simulink model "a1_ex2_sim2"  (R2023a)
settings: Solver=FixedStepAuto  StartTime=0.0  StopTime=30  FixedStep=Ts  RelTol=1e-3
InitFcn:
  | a1_ex2_sim_init
values from neighbouring files (symbols this model uses):
  filter_coeff_bp = firpm(n_bp,fo_bp,ao_bp,w_bp)    [a1_ex2_sim_init.m]
  filter_coeff_lp = firpm(n_lp,fo_lp,ao_lp,w_lp)    [a1_ex2_sim_init.m]
  R = [cos(theta) -sin(theta) 0 ... (first row only)    [a1_ex2_sim_init.m]
  rate_limit_falling = -2    [a1_ex2_sim_init.m]
  rate_limit_rising = 2    [a1_ex2_sim_init.m]
  th1_biceps_left = 0.09    [a1_ex2_sim_init.m]
  th1_biceps_right = 0.09    [a1_ex2_sim_init.m]
  th1_trapezius_left = 0.055    [a1_ex2_sim_init.m]
  th1_trapezius_right = 0.08    [a1_ex2_sim_init.m]
  Ts = 1e-3    (= 0.001)    [a1_ex2_sim_init.m]
libraries: vrlib x1
settings Model: Creator=davide  LastModifiedBy=davide

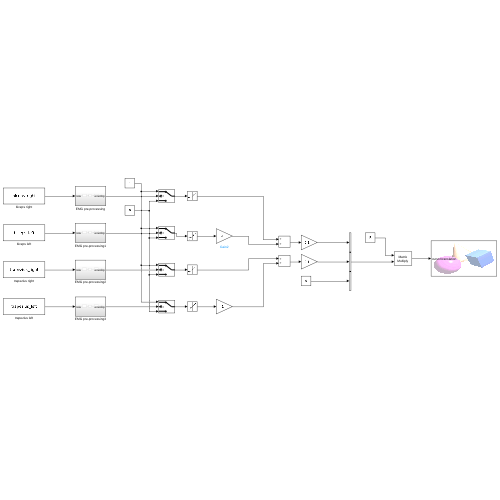
[thumbnail: Simulink's stored preview of the top-level diagram]
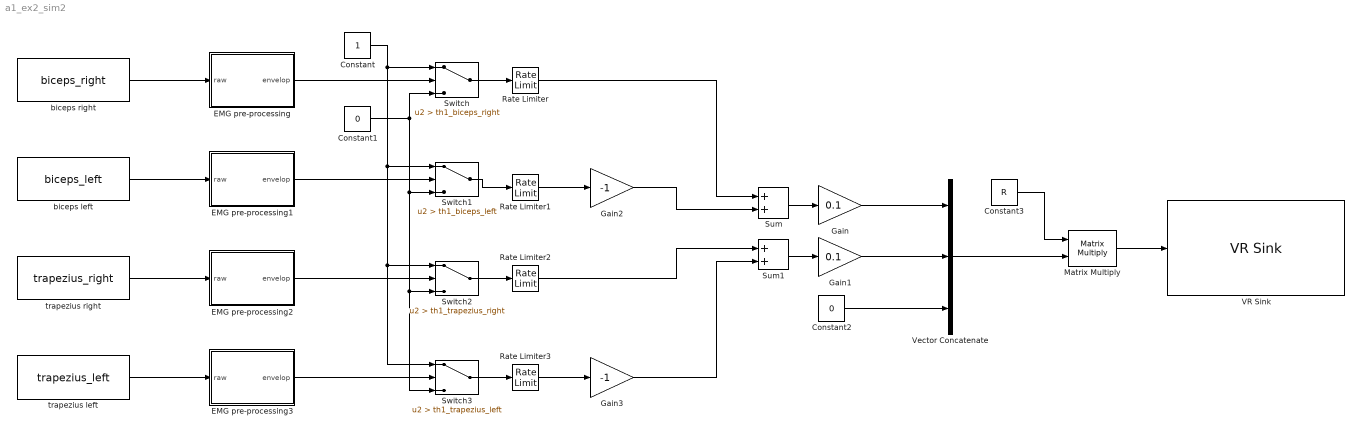
== system a1_ex2_sim2 ==
  Constant : Constant
  Constant1 : Constant  Value=0
  Constant2 : Constant  Value=0
  Constant3 : Constant  Value=R  VectorParams1D=off
  EMG pre-processing : Subsystem
  EMG pre-processing1 : Subsystem
  EMG pre-processing2 : Subsystem
  EMG pre-processing3 : Subsystem
  Gain : Gain  Gain=0.1
  Gain1 : Gain  Gain=0.1
  Gain2 : Gain  Gain=-1
  Gain3 : Gain  Gain=-1
  Matrix Multiply : Product  Multiplication=Matrix(*)
  Rate Limiter{,1..3} (4 alike) : RateLimiter  RisingSlewLimit=rate_limit_rising  FallingSlewLimit=rate_limit_falling  SampleTimeMode=inherited
  Sum : Sum
  Sum1 : Sum
  Switch : Switch  Criteria=u2 > Threshold  Threshold=th1_biceps_right  SaturateOnIntegerOverflow=off  InputSameDT=off
  Switch1 : Switch  Criteria=u2 > Threshold  Threshold=th1_biceps_left  SaturateOnIntegerOverflow=off  InputSameDT=off
  Switch2 : Switch  Criteria=u2 > Threshold  Threshold=th1_trapezius_right  SaturateOnIntegerOverflow=off  InputSameDT=off
  Switch3 : Switch  Criteria=u2 > Threshold  Threshold=th1_trapezius_left  SaturateOnIntegerOverflow=off  InputSameDT=off
  VR Sink : vrlib/VR Sink  InstantiateOnLoad=on  SampleTime=0.1  ViewEnable=on  RemoteChange=off  RemoteView=off  FieldsWritten=cursor.translation.3.1.1.double  WorldFileName=es2_emg/8_palline_color.wrl  AutoView=off  VideoDimensions=[]  AllowVariableSize=off
  Vector Concatenate : Concatenate  NumInputs=3
  biceps left : FromWorkspace  VariableName=biceps_left  OutDataTypeStr=double  SampleTime=Ts
  biceps right : FromWorkspace  VariableName=biceps_right  OutDataTypeStr=double  SampleTime=Ts
  trapezius left : FromWorkspace  VariableName=trapezius_left  OutDataTypeStr=double  SampleTime=Ts
  trapezius right : FromWorkspace  VariableName=trapezius_right  OutDataTypeStr=double  SampleTime=Ts
  wires:
  biceps right/1 -> EMG pre-processing/1(raw)
  biceps left/1 -> EMG pre-processing1/1(raw)
  trapezius right/1 -> EMG pre-processing2/1(raw)
  trapezius left/1 -> EMG pre-processing3/1(raw)
  EMG pre-processing/1(envelop) -> Switch/2
  Constant/1 -> Switch2/1, Switch3/1, Switch1/1, Switch/1
  Constant1/1 -> Switch3/3, Switch2/3, Switch1/3, Switch/3
  Switch/1 -> Rate Limiter/1
  Switch1/1 -> Rate Limiter1/1
  EMG pre-processing1/1(envelop) -> Switch1/2
  EMG pre-processing2/1(envelop) -> Switch2/2
  Switch2/1 -> Rate Limiter2/1
  Switch3/1 -> Rate Limiter3/1
  EMG pre-processing3/1(envelop) -> Switch3/2
  Rate Limiter1/1 -> Gain2/1
  Rate Limiter2/1 -> Sum1/1
  Rate Limiter3/1 -> Gain3/1
  Rate Limiter/1 -> Sum/1
  Gain2/1 -> Sum/2
  Sum/1 -> Gain/1
  Sum1/1 -> Gain1/1
  Gain3/1 -> Sum1/2
  Gain/1 -> Vector Concatenate/1
  Gain1/1 -> Vector Concatenate/2
  Constant3/1 -> Matrix Multiply/1
  Constant2/1 -> Vector Concatenate/3
  Vector Concatenate/1 -> Matrix Multiply/2
  Matrix Multiply/1 -> VR Sink/1

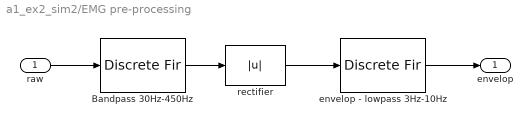
== system a1_ex2_sim2/EMG pre-processing ==
  raw : Inport
  Bandpass 30Hz-450Hz : DiscreteFir  Coefficients=filter_coeff_bp  InputProcessing=Columns as channels (frame based)  SampleTime=Ts
  envelop - lowpass 3Hz-10Hz : DiscreteFir  Coefficients=filter_coeff_lp  InputProcessing=Columns as channels (frame based)  SampleTime=Ts
  rectifier : Abs  SaturateOnIntegerOverflow=off
  envelop : Outport
  wires:
  Bandpass 30Hz-450Hz/1 -> rectifier/1
  rectifier/1 -> envelop - lowpass 3Hz-10Hz/1
  envelop - lowpass 3Hz-10Hz/1 -> envelop/1
  raw/1 -> Bandpass 30Hz-450Hz/1

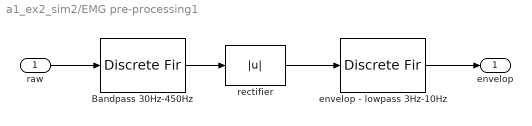
== system a1_ex2_sim2/EMG pre-processing1 ==
  raw : Inport
  Bandpass 30Hz-450Hz : DiscreteFir  Coefficients=filter_coeff_bp  InputProcessing=Columns as channels (frame based)  SampleTime=Ts
  envelop - lowpass 3Hz-10Hz : DiscreteFir  Coefficients=filter_coeff_lp  InputProcessing=Columns as channels (frame based)  SampleTime=Ts
  rectifier : Abs  SaturateOnIntegerOverflow=off
  envelop : Outport
  wires:
  Bandpass 30Hz-450Hz/1 -> rectifier/1
  rectifier/1 -> envelop - lowpass 3Hz-10Hz/1
  envelop - lowpass 3Hz-10Hz/1 -> envelop/1
  raw/1 -> Bandpass 30Hz-450Hz/1

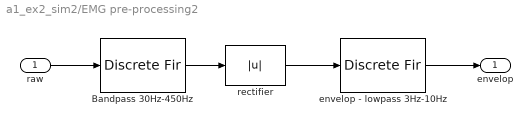
== system a1_ex2_sim2/EMG pre-processing2 ==
  raw : Inport
  Bandpass 30Hz-450Hz : DiscreteFir  Coefficients=filter_coeff_bp  InputProcessing=Columns as channels (frame based)  SampleTime=Ts
  envelop - lowpass 3Hz-10Hz : DiscreteFir  Coefficients=filter_coeff_lp  InputProcessing=Columns as channels (frame based)  SampleTime=Ts
  rectifier : Abs  SaturateOnIntegerOverflow=off
  envelop : Outport
  wires:
  raw/1 -> Bandpass 30Hz-450Hz/1
  envelop - lowpass 3Hz-10Hz/1 -> envelop/1
  rectifier/1 -> envelop - lowpass 3Hz-10Hz/1
  Bandpass 30Hz-450Hz/1 -> rectifier/1

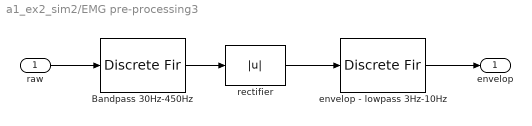
== system a1_ex2_sim2/EMG pre-processing3 ==
  raw : Inport
  Bandpass 30Hz-450Hz : DiscreteFir  Coefficients=filter_coeff_bp  InputProcessing=Columns as channels (frame based)  SampleTime=Ts
  envelop - lowpass 3Hz-10Hz : DiscreteFir  Coefficients=filter_coeff_lp  InputProcessing=Columns as channels (frame based)  SampleTime=Ts
  rectifier : Abs  SaturateOnIntegerOverflow=off
  envelop : Outport
  wires:
  Bandpass 30Hz-450Hz/1 -> rectifier/1
  rectifier/1 -> envelop - lowpass 3Hz-10Hz/1
  envelop - lowpass 3Hz-10Hz/1 -> envelop/1
  raw/1 -> Bandpass 30Hz-450Hz/1
